simulink model "aero_atc"  (R2024a)
settings: Solver=ode45  StartTime=0.0  StopTime=10000  MaxStep=0.25  RelTol=1e-3  EnableMultiTasking=on
PreLoadFcn:
  | aero_atcgui;
InitFcn:
  | aero_init_atc
undefined symbols (not defined in the file): AZ_Sep, BwPw, E, EL_Sep, Lambda, lambda_bp, Loss, Newton, Noise, Pt, rainfall, rainfall_bp, Raphson, Rrange, Rres, sigma_table, SNR, Temp
CloseFcn:
  | h = findobj('Type','figure','Name','Air Traffic RADAR Design Parameters');
  | if ~isempty(h)
  |     close(h);
  | end
Description:
  | Air traffic control demonstration
settings Model: RequirementInfo=9  FPTRunName=Active  Creator=The MathWorks, Inc.  LastModifiedBy=uditpant
settings SolverCC: AlgebraicLoopSolver=TrustRegion  MaxZcPerStep=1
settings DataIOCC: MaxDataPoints=5000  SaveFormat=Array  SaveOutput=off  SignalLogging=off  SaveTime=off  ReturnWorkspaceOutputs=off
settings OptimizationCC: BlockReduction=off  BooleanDataType=off  ExpressionDepthLimit=2147483647  InitFltsAndDblsToZero=on  LifeSpan=inf
settings DebuggingCC: SaveWithParameterizedLinksMsg=none  CheckExecutionContextPreStartOutputMsg=on  SignalResolutionControl=TryResolveAllWithWarning  MultiTaskDSMMsg=warning  MultiTaskCondExecSysMsg=none  FcnCallInpInsideContextMsg=warning  UnconnectedInputMsg=warning  UnconnectedOutputMsg=warning  UnconnectedLineMsg=warning  AllowSymbolicDim=off  StateNameClashWarn=warning  SFUnexpectedBacktrackingDiag=warning  SFNoUnconditionalDefaultTransitionDiag=warning  SFExecutionAtInitializationDiag=none  ArithmeticOperatorsInVariantConditions=warning
settings HardwareCC: ProdBitPerPointer=32  ProdBitPerSizeT=32  ProdBitPerPtrDiffT=32  ProdLargestAtomicFloat=None  ProdIntDivRoundTo=Undefined  ProdEndianess=Unspecified  ProdWordSize=32  ProdHWDeviceType=32-bit Generic
settings ModelReferenceCC: EnableRefExpFcnMdlSchedulingChecks=on  PropagateSignalLabelsOutOfModel=off
settings SFSimCC: SimUseLocalCustomCode=off  SimParseCustomCode=off  CustomCodeUndefinedFunction=UseInterfaceOnly
settings RTWCC: RTWUseLocalCustomCode=off  GPUComputeCapability=3.5  DLArmComputeVersion=19.05
settings CodeAppCC: StateflowObjectComments=on
settings GRTTargetCC: TargetFcnLib=ansi_tfl_tmw.mat  TargetLangStandard=C89/C90 (ANSI)  CombineOutputUpdateFcns=off  GRTInterface=on
settings ConfigComp: CovMetricSettings=d  CovSaveCumulativeToWorkspaceVar=on  CovSaveSingleToWorkspaceVar=on  CovExternalEMLEnable=off  CovSFcnEnable=off

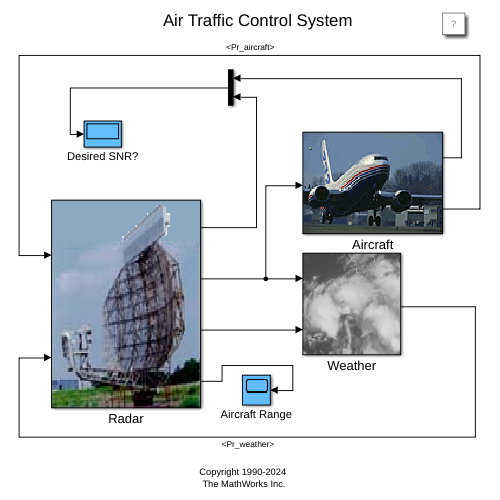
[thumbnail: Simulink's stored preview of the top-level diagram]
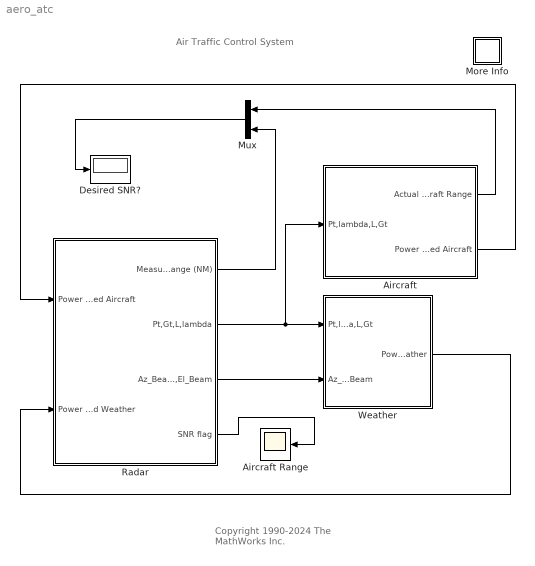
== system aero_atc ==
  note: Copyright 1990-2024
      |  The MathWorks Inc.
  note: Air Traffic Control System
  Aircraft : Subsystem
      mask Display: image('$imagefile'); % Use "Edit Image" on toolstrip to change.
  Aircraft Range : Scope
  Desired SNR? : Display
  More Info : Subsystem
      settings: OpenFcn=showExample('simulink_aerospace/AirTrafficControlRadarDesignExample')
      mask Display: disp('?')
  Mux : Mux  Inputs=2
  Radar : Subsystem
      mask Display: image('$imagefile'); % Use "Edit Image" on toolstrip to change.
  Weather : Subsystem
      mask Display: image('$imagefile'); % Use "Edit Image" on toolstrip to change.
  wires:
  Radar/2(Pt,Gt,L,lambda) -> Aircraft/1(Pt,lambda,L,Gt), Weather/1(Pt,lambda,L,Gt)
  Radar/3(Az_Beam,El_Beam) -> Weather/2(Az_Beam,El_Beam)
  Weather/1(Power Returned Weather) -> Radar/2(Power Received Weather)
  Aircraft/2(Power Returned Aircraft) -> Radar/1(Power Received Aircraft)
  Radar/1(Measured Aircraft Range (NM)) -> Mux/2
  Aircraft/1(Actual Aircraft Range) -> Mux/1
  Mux/1 -> Desired SNR?/1
  Radar/4(SNR flag) -> Aircraft Range/1

== system aero_atc/Aircraft ==
  Pt,lambda,L,Gt : Inport
  Subsystem : Subsystem
  Actual Aircraft Range : Outport  VectorParamsAs1DForOutWhenUnconnected=off
  Power Returned Aircraft : Outport  Port=2  VectorParamsAs1DForOutWhenUnconnected=off
  wires:
  Pt,lambda,L,Gt/1 -> Subsystem/1(Pt,lambda,L,Gt)
  Subsystem/1(Pr_aircraft) -> Power Returned Aircraft/1
  Subsystem/2(Act. Range) -> Actual Aircraft Range/1

== system aero_atc/More Info ==

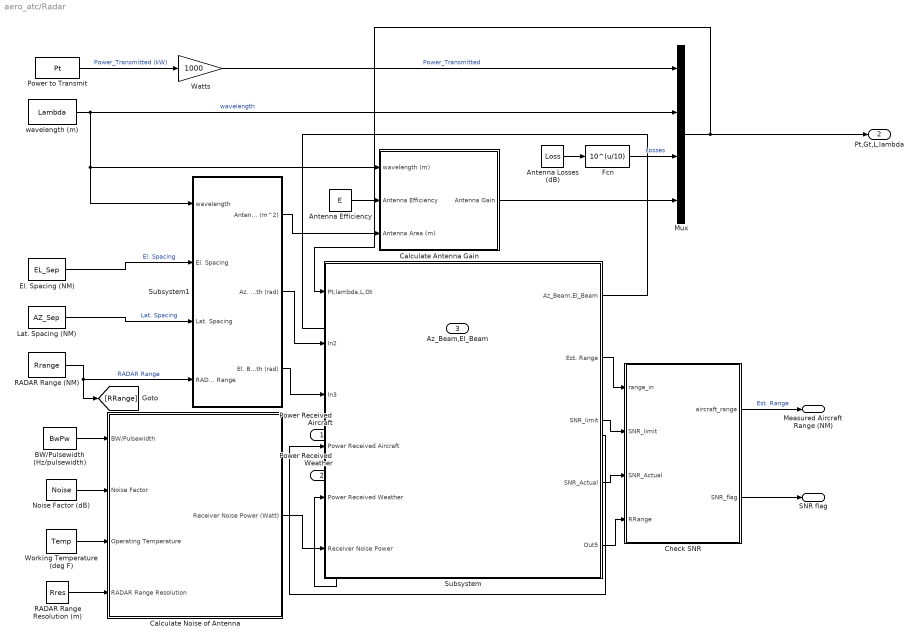
== system aero_atc/Radar ==
  Power Received Aircraft : Inport
  Power Received Weather : Inport  Port=2
  Antenna Efficiency : Constant  Value=E
  Antenna Losses (dB) : Constant  Value=Loss
  BW/Pulsewidth (Hz/pulsewidth) : Constant  Value=BwPw
  Calculate Antenna Gain : Subsystem
  Calculate Noise of Antenna : Subsystem
  Check SNR : Stateflow chart  TreatAsAtomicUnit=on
  El. Spacing (NM) : Constant  Value=EL_Sep
  Fcn : Fcn  Expr=10^(u/10)
  Lat. Spacing (NM) : Constant  Value=AZ_Sep
  Mux : Mux
  Noise Factor (dB) : Constant  Value=Noise
  Power to Transmit : Constant  Value=Pt
  RADAR Range (NM) : Constant  Value=Rrange
  RADAR Range Resolution (m) : Constant  Value=Rres
  Subsystem : Subsystem
  Subsystem1 : Subsystem
  Watts : Gain  Gain=1000  SaturateOnIntegerOverflow=on  OutDataTypeStr=Inherit: Same as input  ParamDataTypeStr=Inherit: Same as input
  Working Temperature (deg F) : Constant  Value=Temp
  "wavelength (m) " : Constant  Value=Lambda
  Measured Aircraft Range (NM) : Outport  VectorParamsAs1DForOutWhenUnconnected=off
  Pt,Gt,L,lambda : Outport  Port=2  VectorParamsAs1DForOutWhenUnconnected=off
  Az_Beam,El_Beam : Outport  Port=3  VectorParamsAs1DForOutWhenUnconnected=off
  SNR flag : Outport  Port=4  VectorParamsAs1DForOutWhenUnconnected=off
  wires:
  Antenna Efficiency/1 -> Calculate Antenna Gain/2(Antenna Efficiency)
  "wavelength (m) "/1 -> Subsystem1/1(wavelength), Calculate Antenna Gain/1(wavelength (m)), Mux/2  "wavelength"
  RADAR Range (NM)/1 -> Subsystem1/4(RADAR Range), [RRange]  "RADAR Range"
  RADAR Range Resolution (m)/1 -> Calculate Noise of Antenna/4(RADAR Range Resolution)
  BW/Pulsewidth (Hz/pulsewidth)/1 -> Calculate Noise of Antenna/1(BW/Pulsewidth)
  Noise Factor (dB)/1 -> Calculate Noise of Antenna/2(Noise Factor)
  Working Temperature (deg F)/1 -> Calculate Noise of Antenna/3(Operating Temperature)
  Mux/1 -> Subsystem/1(Pt,lambda,L,Gt), Pt,Gt,L,lambda/1
  Calculate Antenna Gain/1("Antenna Gain ") -> Mux/4
  Fcn/1 -> Mux/3  "Losses"
  Watts/1 -> Mux/1  "Power_Transmitted"
  Antenna Losses (dB)/1 -> Fcn/1
  Power to Transmit/1 -> Watts/1  "Power_Transmitted (kW)"
  Check SNR/1(aircraft_range) -> Measured Aircraft Range (NM)/1  "Est. Range"
  Check SNR/2(SNR_flag) -> SNR flag/1
  Power Received Aircraft/1 -> Subsystem/4(Power Received Aircraft)
  Power Received Weather/1 -> Subsystem/5(Power Received Weather)
  Calculate Noise of Antenna/1(Receiver Noise Power (Watt)) -> Subsystem/6(Receiver Noise Power)
  Subsystem/1(Az_Beam,El_Beam) -> Az_Beam,El_Beam/1
  Subsystem/2(Est. Range) -> Check SNR/1(range_in)
  Subsystem/3(SNR_limit) -> Check SNR/2(SNR_limit)
  Subsystem/4(SNR_Actual) -> Check SNR/3(SNR_Actual)
  Subsystem/5(Out5) -> Check SNR/4(RRange)
  El. Spacing (NM)/1 -> Subsystem1/2(El. Spacing)  "El. Spacing"
  Lat. Spacing (NM)/1 -> Subsystem1/3(Lat. Spacing)  "Lat. Spacing"
  Subsystem1/1(Antenna Area (m^2)) -> Calculate Antenna Gain/3(Antenna Area (m))
  Subsystem1/2("Az. Beamwidth (rad) ") -> Subsystem/2(In2)
  Subsystem1/3("El. Beamwidth (rad) ") -> Subsystem/3(In3)

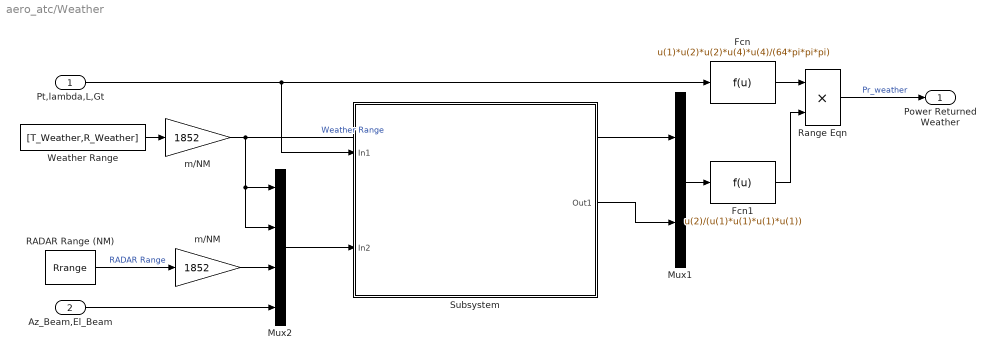
== system aero_atc/Weather ==
  Pt,lambda,L,Gt : Inport
  Az_Beam,El_Beam : Inport  Port=2
  Fcn : Fcn  Expr=u(1)*u(2)*u(2)*u(4)*u(4)/(64*pi*pi*pi)
  Fcn1 : Fcn  Expr=u(2)/(u(1)*u(1)*u(1)*u(1))
  Mux1 : Mux  Inputs=2
  Mux2 : Mux
  RADAR Range (NM) : Constant  Value=Rrange
  Range Eqn : Product  InputSameDT=on  RndMeth=Zero  SaturateOnIntegerOverflow=on  OutDataTypeStr=Inherit: Same as first input
  Subsystem : Subsystem
  Weather Range : FromWorkspace  VariableName=[T_Weather,R_Weather]  Interpolate=off  ZeroCross=off  OutputAfterFinalValue=Holding final value
  m/NM : Gain  Gain=1852  SaturateOnIntegerOverflow=on  OutDataTypeStr=Inherit: Same as input  ParamDataTypeStr=Inherit: Same as input
  "m/NM " : Gain  Gain=1852  SaturateOnIntegerOverflow=on  OutDataTypeStr=Inherit: Same as input  ParamDataTypeStr=Inherit: Same as input
  Power Returned Weather : Outport  VectorParamsAs1DForOutWhenUnconnected=off
  wires:
  m/NM/1 -> Mux2/3
  RADAR Range (NM)/1 -> m/NM/1  "RADAR Range"
  Az_Beam,El_Beam/1 -> Mux2/4
  "m/NM "/1 -> Mux1/1, Mux2/1, Mux2/2  "Weather Range"
  Mux1/1 -> Fcn1/1
  Weather Range/1 -> "m/NM "/1
  Pt,lambda,L,Gt/1 -> Fcn/1, Subsystem/1(In1)
  Fcn1/1 -> Range Eqn/2
  Fcn/1 -> Range Eqn/1
  Range Eqn/1 -> Power Returned Weather/1  "Pr_weather"
  Mux2/1 -> Subsystem/2(In2)
  Subsystem/1(Out1) -> Mux1/2

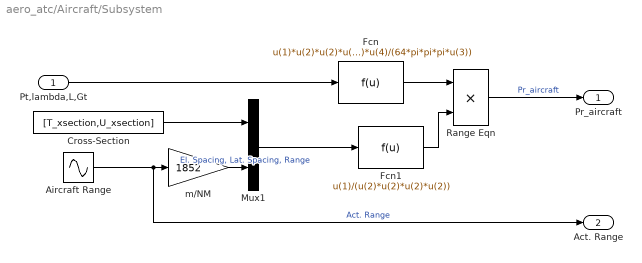
== system aero_atc/Aircraft/Subsystem ==
  Pt,lambda,L,Gt : Inport
  Aircraft Range : Sin  Amplitude=25  Bias=35  Frequency=0.0025  SampleTime=0
  Cross-Section : FromWorkspace  VariableName=[T_xsection,U_xsection]  Interpolate=off  ZeroCross=off  OutputAfterFinalValue=Holding final value
  Fcn : Fcn  Expr=u(1)*u(2)*u(2)*u(4)*u(4)/(64*pi*pi*pi*u(3))
  Fcn1 : Fcn  Expr=u(1)/(u(2)*u(2)*u(2)*u(2))
  Mux1 : Mux  Inputs=2
  Range Eqn : Product  InputSameDT=on  RndMeth=Zero  SaturateOnIntegerOverflow=on  OutDataTypeStr=Inherit: Same as first input
  m/NM : Gain  Gain=1852  SaturateOnIntegerOverflow=on  OutDataTypeStr=Inherit: Same as input  ParamDataTypeStr=Inherit: Same as input
  Pr_aircraft : Outport
  Act. Range : Outport  Port=2
  wires:
  Pt,lambda,L,Gt/1 -> Fcn/1
  Mux1/1 -> Fcn1/1
  m/NM/1 -> Mux1/2  "El. Spacing, Lat. Spacing, Range"
  Fcn1/1 -> Range Eqn/2
  Aircraft Range/1 -> Act. Range/1, m/NM/1  "Act. Range"
  Cross-Section/1 -> Mux1/1
  Fcn/1 -> Range Eqn/1
  Range Eqn/1 -> Pr_aircraft/1  "Pr_aircraft"

== system aero_atc/Radar/Calculate Antenna Gain ==
  wavelength (m) : Inport
  Antenna Efficiency : Inport  Port=2
  Antenna Area (m) : Inport  Port=3
  Subsystem : Subsystem
  "Antenna Gain " : Outport  VectorParamsAs1DForOutWhenUnconnected=off
  wires:
  wavelength (m)/1 -> Subsystem/1(wavelength (m))
  Antenna Efficiency/1 -> Subsystem/2(Antenna Efficiency)
  Antenna Area (m)/1 -> Subsystem/3(Antenna Area (m))
  Subsystem/1(Gain) -> "Antenna Gain "/1

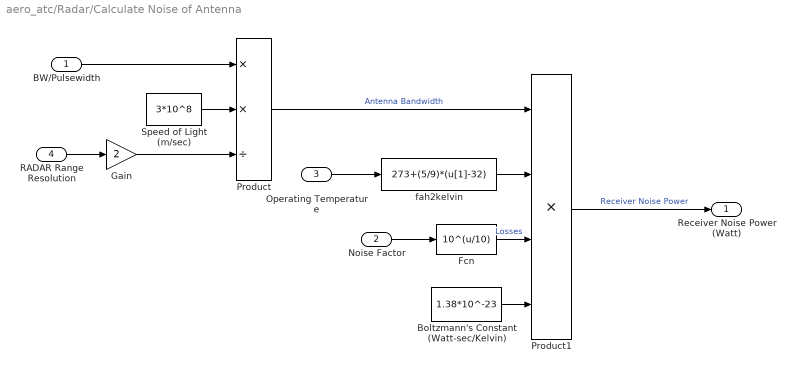
== system aero_atc/Radar/Calculate Noise of Antenna ==
  BW/Pulsewidth : Inport
  Noise Factor : Inport  Port=2
  Operating Temperature : Inport  Port=3
  RADAR Range Resolution : Inport  Port=4
  Boltzmann's Constant (Watt-sec/Kelvin) : Constant  Value=1.38*10^-23
  Fcn : Fcn  Expr=10^(u/10)
  Gain : Gain  Gain=2  SaturateOnIntegerOverflow=on  OutDataTypeStr=Inherit: Same as input  ParamDataTypeStr=Inherit: Same as input
  Product : Product  Inputs=**/  InputSameDT=on  RndMeth=Zero  SaturateOnIntegerOverflow=on  OutDataTypeStr=Inherit: Same as first input
  Product1 : Product  Inputs=4  InputSameDT=on  RndMeth=Zero  SaturateOnIntegerOverflow=on  OutDataTypeStr=Inherit: Same as first input
  Speed of Light (m/sec) : Constant  Value=3*10^8
  fah2kelvin : Fcn  Expr=273+(5/9)*(u[1]-32)
  Receiver Noise Power (Watt) : Outport  VectorParamsAs1DForOutWhenUnconnected=off
  wires:
  Speed of Light (m/sec)/1 -> Product/2
  Gain/1 -> Product/3
  BW/Pulsewidth/1 -> Product/1
  RADAR Range Resolution/1 -> Gain/1
  Product/1 -> Product1/1  "Antenna Bandwidth"
  fah2kelvin/1 -> Product1/2
  Boltzmann's Constant (Watt-sec/Kelvin)/1 -> Product1/4
  Product1/1 -> Receiver Noise Power (Watt)/1  "Receiver Noise Power"
  Noise Factor/1 -> Fcn/1
  Fcn/1 -> Product1/3  "Losses"
  Operating Temperature/1 -> fah2kelvin/1

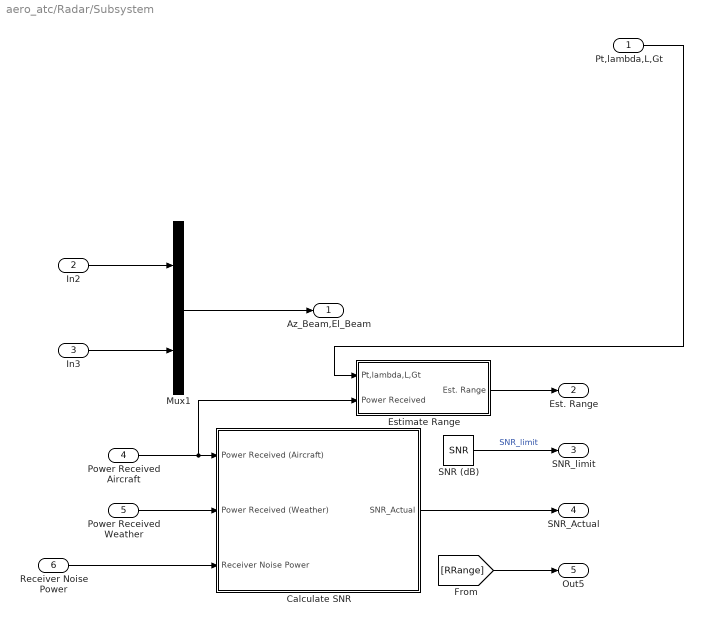
== system aero_atc/Radar/Subsystem ==
  Pt,lambda,L,Gt : Inport
  In2 : Inport  Port=2
  In3 : Inport  Port=3
  Power Received Aircraft : Inport  Port=4
  Power Received Weather : Inport  Port=5
  Receiver Noise Power : Inport  Port=6
  Calculate SNR : Subsystem
  Estimate Range : Subsystem
  Mux1 : Mux  Inputs=2
  SNR (dB) : Constant  Value=SNR
  Az_Beam,El_Beam : Outport  VectorParamsAs1DForOutWhenUnconnected=off
  Est. Range : Outport  Port=2
  SNR_limit : Outport  Port=3
  SNR_Actual : Outport  Port=4
  Out5 : Outport  Port=5
  wires:
  Power Received Weather/1 -> Calculate SNR/2(Power Received (Weather))
  Calculate SNR/1(SNR_Actual) -> SNR_Actual/1
  Mux1/1 -> Az_Beam,El_Beam/1
  Estimate Range/1(Est. Range) -> Est. Range/1
  Power Received Aircraft/1 -> Calculate SNR/1(Power Received (Aircraft)), Estimate Range/2(Power Received)
  SNR (dB)/1 -> SNR_limit/1  "SNR_limit"
  [RRange] -> Out5/1
  In2/1 -> Mux1/1
  Pt,lambda,L,Gt/1 -> Estimate Range/1(Pt,lambda,L,Gt)
  In3/1 -> Mux1/2
  Receiver Noise Power/1 -> Calculate SNR/3(Receiver Noise Power)

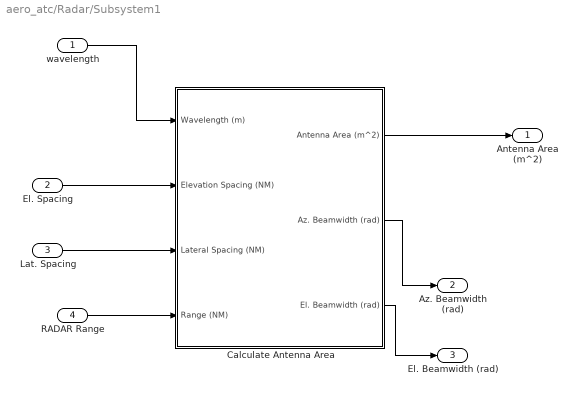
== system aero_atc/Radar/Subsystem1 ==
  wavelength : Inport
  El. Spacing : Inport  Port=2
  Lat. Spacing : Inport  Port=3
  RADAR Range : Inport  Port=4
  Calculate Antenna Area : Subsystem
  Antenna Area (m^2) : Outport
  "Az. Beamwidth (rad) " : Outport  Port=2
  "El. Beamwidth (rad) " : Outport  Port=3
  wires:
  RADAR Range/1 -> Calculate Antenna Area/4(Range (NM))
  wavelength/1 -> Calculate Antenna Area/1(Wavelength (m))
  Calculate Antenna Area/3("El. Beamwidth (rad) ") -> "El. Beamwidth (rad) "/1
  Calculate Antenna Area/1(Antenna Area (m^2)) -> Antenna Area (m^2)/1
  Lat. Spacing/1 -> Calculate Antenna Area/3(Lateral Spacing (NM))
  El. Spacing/1 -> Calculate Antenna Area/2(Elevation Spacing (NM))
  Calculate Antenna Area/2("Az. Beamwidth (rad) ") -> "Az. Beamwidth (rad) "/1

== system aero_atc/Weather/Subsystem ==
  In1 : Inport
  In2 : Inport  Port=2
  Subsystem : Subsystem
  Out1 : Outport
  wires:
  In1/1 -> Subsystem/1(In1)
  In2/1 -> Subsystem/2(In2)
  Subsystem/1(Out1) -> Out1/1

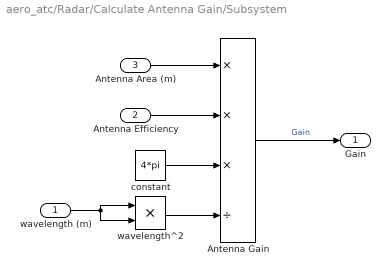
== system aero_atc/Radar/Calculate Antenna Gain/Subsystem ==
  wavelength (m) : Inport
  Antenna Efficiency : Inport  Port=2
  Antenna Area (m) : Inport  Port=3
  Antenna Gain : Product  Inputs=***/  InputSameDT=on  RndMeth=Zero  SaturateOnIntegerOverflow=on  OutDataTypeStr=Inherit: Same as first input
  constant : Constant  Value=4*pi
  wavelength^2 : Product  InputSameDT=on  RndMeth=Zero  SaturateOnIntegerOverflow=on  OutDataTypeStr=Inherit: Same as first input
  Gain : Outport
  wires:
  wavelength^2/1 -> Antenna Gain/4
  Antenna Efficiency/1 -> Antenna Gain/2
  wavelength (m)/1 -> wavelength^2/2, wavelength^2/1
  Antenna Area (m)/1 -> Antenna Gain/1
  constant/1 -> Antenna Gain/3
  Antenna Gain/1 -> Gain/1  "Gain"

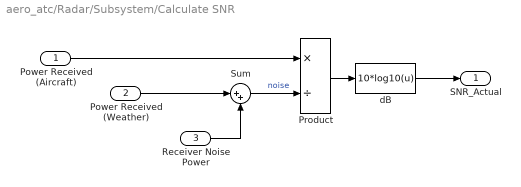
== system aero_atc/Radar/Subsystem/Calculate SNR ==
  Power Received (Aircraft) : Inport
  Power Received (Weather) : Inport  Port=2
  Receiver Noise Power : Inport  Port=3
  Product : Product  Inputs=*/  InputSameDT=on  RndMeth=Zero  SaturateOnIntegerOverflow=on  OutDataTypeStr=Inherit: Same as first input
  Sum : Sum  Inputs=|++  InputSameDT=on  SaturateOnIntegerOverflow=on  OutDataTypeStr=Inherit: Same as first input
  dB : Fcn  Expr=10*log10(u)
  SNR_Actual : Outport  VectorParamsAs1DForOutWhenUnconnected=off
  wires:
  Sum/1 -> Product/2  "noise"
  Power Received (Aircraft)/1 -> Product/1
  Power Received (Weather)/1 -> Sum/1
  Receiver Noise Power/1 -> Sum/2
  Product/1 -> dB/1
  dB/1 -> SNR_Actual/1

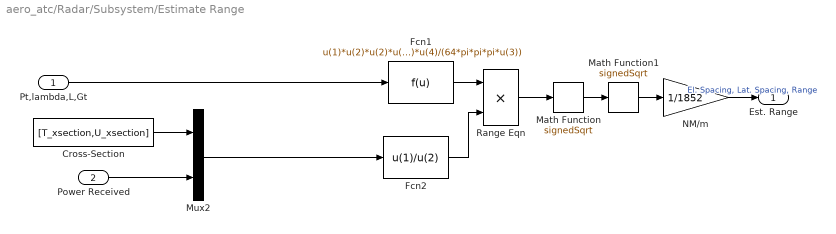
== system aero_atc/Radar/Subsystem/Estimate Range ==
  Pt,lambda,L,Gt : Inport
  Power Received : Inport  Port=2
  Cross-Section : FromWorkspace  VariableName=[T_xsection,U_xsection]  ZeroCross=off
  Fcn1 : Fcn  Expr=u(1)*u(2)*u(2)*u(4)*u(4)/(64*pi*pi*pi*u(3))
  Fcn2 : Fcn  Expr=u(1)/u(2)
  Math Function : Sqrt  Operator=signedSqrt  AlgorithmType=Newton-Raphson
  Math Function1 : Sqrt  Operator=signedSqrt  AlgorithmType=Newton-Raphson
  Mux2 : Mux  Inputs=2
  NM/m : Gain  Gain=1/1852  SaturateOnIntegerOverflow=on  OutDataTypeStr=Inherit: Same as input  ParamDataTypeStr=Inherit: Same as input
  Range Eqn : Product  InputSameDT=on  RndMeth=Zero  SaturateOnIntegerOverflow=on  OutDataTypeStr=Inherit: Same as first input
  Est. Range : Outport  VectorParamsAs1DForOutWhenUnconnected=off
  wires:
  Pt,lambda,L,Gt/1 -> Fcn1/1
  Fcn1/1 -> Range Eqn/1
  Fcn2/1 -> Range Eqn/2
  Range Eqn/1 -> Math Function/1
  Math Function/1 -> Math Function1/1
  Math Function1/1 -> NM/m/1
  NM/m/1 -> Est. Range/1  "El. Spacing, Lat. Spacing, Range"
  Cross-Section/1 -> Mux2/1
  Power Received/1 -> Mux2/2
  Mux2/1 -> Fcn2/1

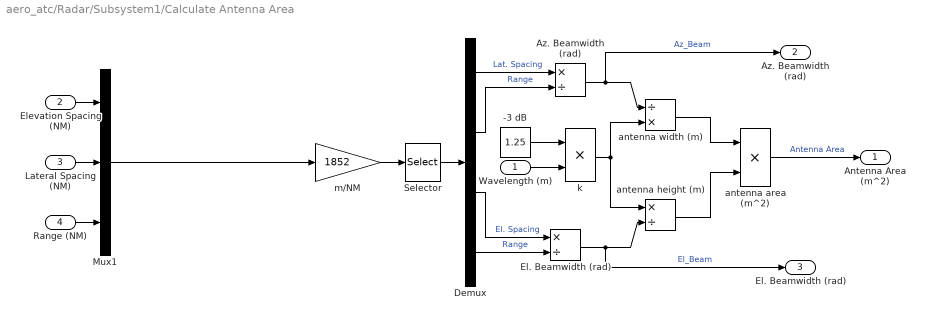
== system aero_atc/Radar/Subsystem1/Calculate Antenna Area ==
  Wavelength (m) : Inport
  Elevation Spacing (NM) : Inport  Port=2
  Lateral Spacing (NM) : Inport  Port=3
  Range (NM) : Inport  Port=4
  "-3 dB  " : Constant  Value=1.25
  Az. Beamwidth (rad) : Product  Inputs=*/  InputSameDT=on  RndMeth=Zero  SaturateOnIntegerOverflow=on  OutDataTypeStr=Inherit: Same as first input
  Demux : Demux
      settings: DisplayOption=none
  El. Beamwidth (rad) : Product  Inputs=*/  InputSameDT=on  RndMeth=Zero  SaturateOnIntegerOverflow=on  OutDataTypeStr=Inherit: Same as first input
  Mux1 : Mux  Inputs=3
  Selector : Selector  InputPortWidth=3  IndexOptions=Index vector (dialog)  Indices=[1 3 2 3]  OutputSizes=1
  antenna area (m^2) : Product  InputSameDT=on  RndMeth=Zero  SaturateOnIntegerOverflow=on  OutDataTypeStr=Inherit: Same as first input
  antenna height (m) : Product  Inputs=*/  InputSameDT=on  RndMeth=Zero  SaturateOnIntegerOverflow=on  OutDataTypeStr=Inherit: Same as first input
  antenna width (m) : Product  Inputs=/*  InputSameDT=on  RndMeth=Zero  SaturateOnIntegerOverflow=on  OutDataTypeStr=Inherit: Same as first input
  k : Product  Inputs=**  InputSameDT=on  RndMeth=Zero  SaturateOnIntegerOverflow=on  OutDataTypeStr=Inherit: Same as first input
  m/NM : Gain  Gain=1852  SaturateOnIntegerOverflow=on  OutDataTypeStr=Inherit: Same as input  ParamDataTypeStr=Inherit: Same as input
  Antenna Area (m^2) : Outport  VectorParamsAs1DForOutWhenUnconnected=off
  "Az. Beamwidth (rad) " : Outport  Port=2  VectorParamsAs1DForOutWhenUnconnected=off
  "El. Beamwidth (rad) " : Outport  Port=3  VectorParamsAs1DForOutWhenUnconnected=off
  wires:
  m/NM/1 -> Selector/1
  Selector/1 -> Demux/1
  Demux/1 -> Az. Beamwidth (rad)/1  "Lat. Spacing"
  Demux/2 -> Az. Beamwidth (rad)/2  "Range"
  Demux/3 -> El. Beamwidth (rad)/1  "El. Spacing"
  Demux/4 -> El. Beamwidth (rad)/2  "Range"
  Wavelength (m)/1 -> k/2
  "-3 dB  "/1 -> k/1
  k/1 -> antenna height (m)/1, antenna width (m)/2
  Az. Beamwidth (rad)/1 -> antenna width (m)/1, "Az. Beamwidth (rad) "/1  "Az_Beam"
  antenna width (m)/1 -> antenna area (m^2)/1
  antenna height (m)/1 -> antenna area (m^2)/2
  antenna area (m^2)/1 -> Antenna Area (m^2)/1  "Antenna Area"
  El. Beamwidth (rad)/1 -> antenna height (m)/2, "El. Beamwidth (rad) "/1  "El_Beam"
  Mux1/1 -> m/NM/1
  Elevation Spacing (NM)/1 -> Mux1/1
  Lateral Spacing (NM)/1 -> Mux1/2
  Range (NM)/1 -> Mux1/3

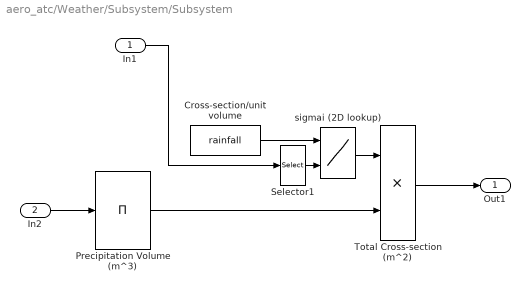
== system aero_atc/Weather/Subsystem/Subsystem ==
  In1 : Inport
  In2 : Inport  Port=2
  Cross-section/unit volume : Constant  Value=rainfall
  Precipitation Volume (m^3) : Product  Inputs=*  InputSameDT=on  RndMeth=Zero  SaturateOnIntegerOverflow=on  OutDataTypeStr=Inherit: Same as first input
  Selector1 : Selector  InputPortWidth=4  IndexOptions=Index vector (dialog)  Indices=2  OutputSizes=1
  Total Cross-section (m^2) : Product  InputSameDT=on  RndMeth=Zero  SaturateOnIntegerOverflow=on  OutDataTypeStr=Inherit: Same as first input
  sigmai (2D lookup) : Lookup_n-D  BreakpointsForDimension1=rainfall_bp  BreakpointsForDimension2=lambda_bp  Table=sigma_table  SaturateOnIntegerOverflow=on
      settings: InputPortMap=u0,u1
  Out1 : Outport
  wires:
  In1/1 -> Selector1/1
  sigmai (2D lookup)/1 -> Total Cross-section (m^2)/1
  Selector1/1 -> sigmai (2D lookup)/2
  Cross-section/unit volume/1 -> sigmai (2D lookup)/1
  Total Cross-section (m^2)/1 -> Out1/1
  Precipitation Volume (m^3)/1 -> Total Cross-section (m^2)/2
  In2/1 -> Precipitation Volume (m^3)/1

== stateflow chart aero_atc/Radar/Check SNR ==
  settings: updateMethod=CONTINUOUS
  state Visibility [parallel]
    settings: executionOrder=1
    state ?
      state detect
        during: aircraft_range = range_in;
      state no_detect
        during: aircraft_range =0;
      no_detect -> detect : [(SNR_Actual > 6) && (range_in <= RRange)]
          | { aircraft_range = range_in;}
      detect -> no_detect : [(SNR_Actual <= 6) || (range_in > RRange)]
          | { aircraft_range = 0;}
    (default) -> (junction 17)
    (junction 17) -> no_detect [order 1] : [(SNR_Actual <= 6) || (range_in > RRange)]
        | { aircraft_range =0;}
    (junction 17) -> detect [order 2] : %(SNR_Actual > 6) && (range_in <= RRange)
        | { aircraft_range = range_in;}
  state SNR [parallel]
    settings: executionOrder=2
    state Less_than
    state Equal_to_or_Greater_than
    (default) -> (junction 18)
    (junction 18) -> Less_than [order 2] : %SNR_Actual < SNR_limit
        | {SNR_flag = 0;}
    (junction 18) -> Equal_to_or_Greater_than [order 1] : [SNR_Actual >= SNR_limit]{SNR_flag = 1;}
    Less_than -> Equal_to_or_Greater_than : [SNR_Actual >= SNR_limit]{SNR_flag = 1;}
    Equal_to_or_Greater_than -> Less_than : [SNR_Actual < SNR_limit]{SNR_flag = 0;}
  data: range_in input double size=1; SNR_limit input double size=1; SNR_Actual input double size=1; aircraft_range output double size=1 =0; RRange input double size=1; SNR_flag output double size=1
